simulink model "SFusion"  (Simulink 9.2)
settings: Solver=FixedStepAuto  StartTime=0.0  StopTime=inf  FixedStep=0.01  RelTol=1e-3  EnableMultiTasking=on
values from neighbouring files (symbols this model uses):
  CLOCK_SEL_PLL = uint8(hex2dec('01'))    [Sfusion.m]
  PWR_MGMNT_1 = uint8(hex2dec('6B'))    [Sfusion.m]
undefined symbols (not defined in the file or in its folder): BIT_H_RESET, BITS_DLPF_CFG_188HZ, BITS_FS_250DPS, BITS_FS_2G, Init, Initialize, MPUREG_ACCEL_CONFIG, MPUREG_GYRO_CONFIG, MPUREG_GYRO_XOUT_H, READ_FLAG
libraries: mbedblockslib x22, arduinolib x20, simulink x15
settings Model: Creator=Syed Imtiaz Ali Shah  LastModifiedBy=Syed Imtiaz Ali Shah  SimulationMode=external  ExtModeTrigDuration=2
settings DataIOCC: LimitDataPoints=off  SaveFormat=Dataset  SignalLoggingSaveFormat=Dataset
settings OptimizationCC: EnhancedBackFolding=on  PassReuseOutputArgsAs=Individual arguments  LifeSpan=auto  MaxStackSize=64  OptimizeBlockOrder=speed  DifferentSizesBufferReuse=on  OptimizationCustomize=off
settings DebuggingCC: UnderspecifiedInitializationDetection=Simplified  MergeDetectMultiDrivingBlocksExec=error  ParameterTunabilityLossMsg=error  FcnCallInpInsideContextMsg=error  StateNameClashWarn=none  SFUnexpectedBacktrackingDiag=error  SFNoUnconditionalDefaultTransitionDiag=error  SFExecutionAtInitializationDiag=warning
settings HardwareCC: ProdBitPerInt=16  ProdBitPerPointer=16  ProdBitPerSizeT=16  ProdBitPerPtrDiffT=16  ProdIntDivRoundTo=Zero  ProdEndianess=LittleEndian  ProdWordSize=8  ProdHWDeviceType=Atmel->AVR
settings ModelReferenceCC: PropagateSignalLabelsOutOfModel=on
settings SFSimCC: SimUseLocalCustomCode=on  MATLABDynamicMemAlloc=off
settings RTWCC: SystemTargetFile=ert.tlc  HardwareBoard=Arduino Mega 2560  TLCOptions=-aInlineSetEventsForThisBaseRateFcn=TLC_FALSE -aSuppressMultiTaskScheduler=TLC_FALSE -aRateBasedStepFcn=1  TemplateMakefile=ert_default_tmf  Description=Embedded Coder  GenerateReport=on  RTWUseLocalCustomCode=on  Toolchain=Arduino AVR  BuildConfiguration=Faster Runs  IncludeHyperlinkInReport=on  LaunchReport=on  GenerateTraceInfo=on  GenerateTraceReport=on  GenerateTraceReportSl=on  GenerateTraceReportSf=on  GenerateTraceReportEml=on
settings MATStruct: className=codertarget.tools.BuildHook  argsTopModelOnly=[]  excludedModels=[]  includeReferencedModels=on  includeTopModel=on  enabled=on  UseCoderTarget=[1]  TargetHardware=Arduino Mega 2560  RTOS=Baremetal  Scheduler_interrupt_source=[0.0]  DataVersion=2016.02  IPAddress=codertarget.arduinobase.registry.getLoopbackIP;  Port=17725  Verbose=[0]  Configuration=Serial  COMPortBaud=921600  BuildAction=Build, load and run  Set_host_COM_port=Manually  COM_port_number=4  Enable_SimulinkIO=[1.0]  Enable_overrun_detection=[0.0]  Digital_output_to_set_on_overrun=13  Analog_input_reference_voltage=[0.0]  Serial0_baud_rate=9600  Serial1_baud_rate=9600  Serial2_baud_rate=9600  Serial3_baud_rate=9600  I2C0BusSpeedHz=100000  SPI_clock_out_frequency=1000  SPI_mode=Mode 0 - Clock Polarity 0, Clock Phase 0  SPI_bitorder=MSB first  Disable_DHCP_Ethernet=[0.0]  Local_ip_address=192.168.0.20  Local_mac_address=DE:AD:BE:EF:FE:ED  Wifi_Hardware=WiFi shield  Disable_DHCP_Wifi=[0.0]  Wifi_ip_address=192.168.1.20  Wifi_SSID=yourNetwork  Set_Wifi_Encryption=None  Wifi_WEP_key=D0D0DEADF00DABBADEAFBEADED  Wifi_WEP_key_index=0  Wifi_WPA_password=secretPassword  Wifi_ESP8266_HW_serial_port=Serial 0  Enable_CustomServer=0  IP_address=184.106.153.149
settings CodeAppCC: ForceParamTrailComments=on  IgnoreCustomStorageClasses=off  OperatorAnnotations=on  SimulinkDataObjDesc=on  SFDataObjDesc=on  InsertBlockDesc=on  StateflowObjectComments=off
settings ERTTargetCC: SupportContinuousTime=on  SupportVariableSizeSignals=on
settings ConfigComp: CovMetricSettings=dwe  CovHtmlReporting=off  CovSaveCumulativeToWorkspaceVar=off  CovSaveSingleToWorkspaceVar=off  CovExternalEMLEnable=on

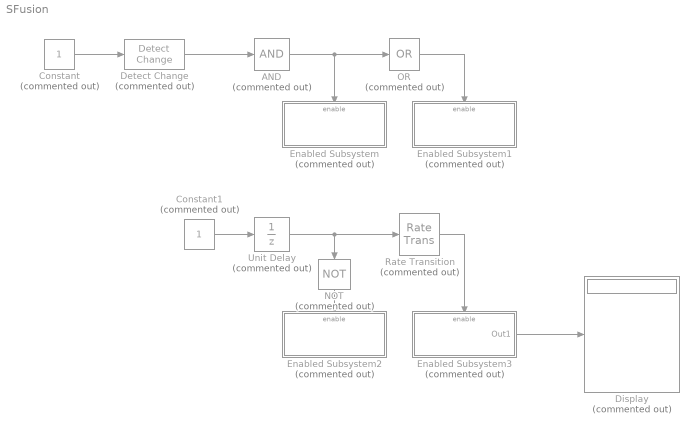
== system SFusion ==
  AND : Logic  Commented=on  Inputs=1  AllPortsSameDT=off  OutDataTypeStr=boolean
  Constant : Constant  Commented=on
  Constant1 : Constant  Commented=on
  Detect Change : simulink/Logic and Bit Operations/Detect Change  Commented=on  vinit=0  OutDataTypeStr=boolean
  Display : Display  Commented=on
  Enabled Subsystem : Subsystem  Commented=on  TreatAsAtomicUnit=on
  Enabled Subsystem1 : Subsystem  Commented=on  TreatAsAtomicUnit=on
  Enabled Subsystem2 : Subsystem  Commented=on  TreatAsAtomicUnit=on
  Enabled Subsystem3 : Subsystem  Commented=on  TreatAsAtomicUnit=on
  NOT : Logic  Commented=on  Operator=NOT  AllPortsSameDT=off  OutDataTypeStr=boolean
  OR : Logic  Commented=on  Operator=OR  Inputs=1  AllPortsSameDT=off  OutDataTypeStr=boolean
  Rate Transition : RateTransition  Commented=on
  Unit Delay : UnitDelay  Commented=on  SampleTime=-1
  wires:
  Constant/1 -> Detect Change/1
  Detect Change/1 -> AND/1
  AND/1 -> OR/1, Enabled Subsystem/Enable
  OR/1 -> Enabled Subsystem1/Enable
  Constant1/1 -> Unit Delay/1
  NOT/1 -> Enabled Subsystem2/Enable
  Unit Delay/1 -> NOT/1, Rate Transition/1
  Rate Transition/1 -> Enabled Subsystem3/Enable
  Enabled Subsystem3/1(Out1) -> Display/1

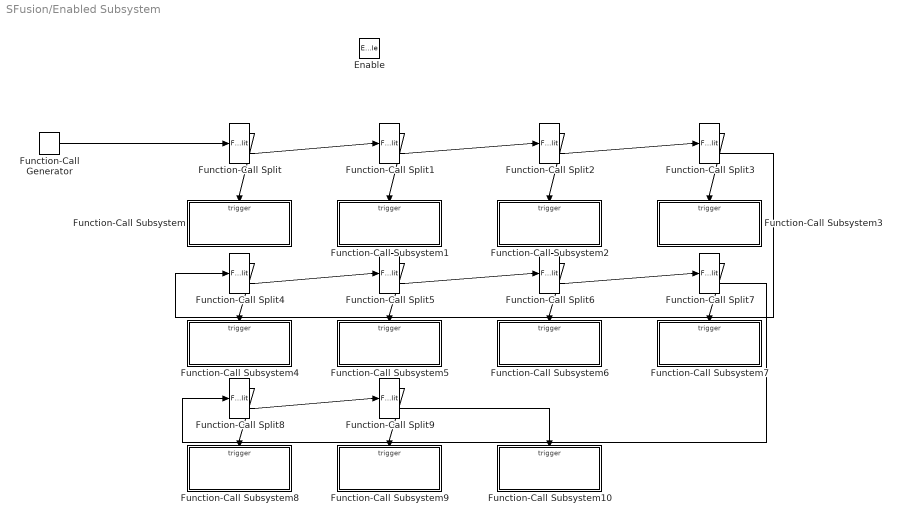
== system SFusion/Enabled Subsystem ==
  Enable : EnablePort
  Function-Call Generator : simulink/Ports & Subsystems/Function-Call Generator  sample_time=1  numberOfIterations=1
  Function-Call Split{,1..9} (10 alike) : FunctionCallSplit  NumOutputPorts=2
  Function-Call Subsystem : Subsystem  TreatAsAtomicUnit=on
  Function-Call Subsystem1 : Subsystem  TreatAsAtomicUnit=on
  Function-Call Subsystem10 : Subsystem  TreatAsAtomicUnit=on
  Function-Call Subsystem2 : Subsystem  TreatAsAtomicUnit=on
  Function-Call Subsystem3 : Subsystem  TreatAsAtomicUnit=on
  Function-Call Subsystem4 : Subsystem  TreatAsAtomicUnit=on
  Function-Call Subsystem5 : Subsystem  TreatAsAtomicUnit=on
  Function-Call Subsystem6 : Subsystem  TreatAsAtomicUnit=on
  Function-Call Subsystem7 : Subsystem  TreatAsAtomicUnit=on
  Function-Call Subsystem8 : Subsystem  TreatAsAtomicUnit=on
  Function-Call Subsystem9 : Subsystem  TreatAsAtomicUnit=on
  wires:
  Function-Call Split/1 -> Function-Call Subsystem/Trigger
  Function-Call Split/2 -> Function-Call Split1/1
  Function-Call Split7/1 -> Function-Call Subsystem7/Trigger
  Function-Call Split8/1 -> Function-Call Subsystem8/Trigger
  Function-Call Split9/2 -> Function-Call Subsystem10/Trigger
  Function-Call Split8/2 -> Function-Call Split9/1
  Function-Call Split9/1 -> Function-Call Subsystem9/Trigger
  Function-Call Split5/2 -> Function-Call Split6/1
  Function-Call Split6/1 -> Function-Call Subsystem6/Trigger
  Function-Call Split5/1 -> Function-Call Subsystem5/Trigger
  Function-Call Split4/1 -> Function-Call Subsystem4/Trigger
  Function-Call Split4/2 -> Function-Call Split5/1
  Function-Call Split3/2 -> Function-Call Split4/1
  Function-Call Split6/2 -> Function-Call Split7/1
  Function-Call Split7/2 -> Function-Call Split8/1
  Function-Call Split1/1 -> Function-Call Subsystem1/Trigger
  Function-Call Split1/2 -> Function-Call Split2/1
  Function-Call Split2/1 -> Function-Call Subsystem2/Trigger
  Function-Call Split2/2 -> Function-Call Split3/1
  Function-Call Split3/1 -> Function-Call Subsystem3/Trigger
  Function-Call Generator/1 -> Function-Call Split/1

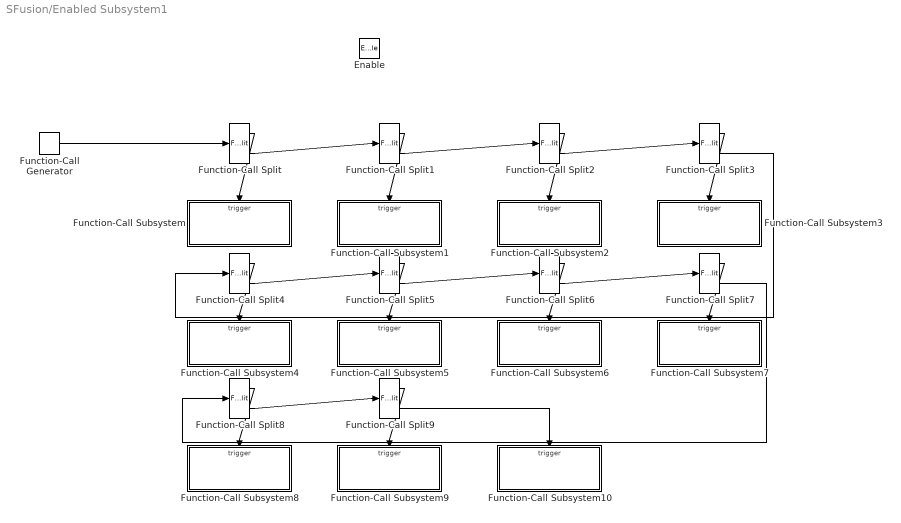
== system SFusion/Enabled Subsystem1 ==
  Enable : EnablePort
  Function-Call Generator : simulink/Ports & Subsystems/Function-Call Generator  sample_time=1  numberOfIterations=1
  Function-Call Split{,1..9} (10 alike) : FunctionCallSplit  NumOutputPorts=2
  Function-Call Subsystem : Subsystem  TreatAsAtomicUnit=on
  Function-Call Subsystem1 : Subsystem  TreatAsAtomicUnit=on
  Function-Call Subsystem10 : Subsystem  TreatAsAtomicUnit=on
  Function-Call Subsystem2 : Subsystem  TreatAsAtomicUnit=on
  Function-Call Subsystem3 : Subsystem  TreatAsAtomicUnit=on
  Function-Call Subsystem4 : Subsystem  TreatAsAtomicUnit=on
  Function-Call Subsystem5 : Subsystem  TreatAsAtomicUnit=on
  Function-Call Subsystem6 : Subsystem  TreatAsAtomicUnit=on
  Function-Call Subsystem7 : Subsystem  TreatAsAtomicUnit=on
  Function-Call Subsystem8 : Subsystem  TreatAsAtomicUnit=on
  Function-Call Subsystem9 : Subsystem  TreatAsAtomicUnit=on
  wires:
  Function-Call Generator/1 -> Function-Call Split/1
  Function-Call Split3/1 -> Function-Call Subsystem3/Trigger
  Function-Call Split2/2 -> Function-Call Split3/1
  Function-Call Split2/1 -> Function-Call Subsystem2/Trigger
  Function-Call Split1/2 -> Function-Call Split2/1
  Function-Call Split1/1 -> Function-Call Subsystem1/Trigger
  Function-Call Split7/2 -> Function-Call Split8/1
  Function-Call Split6/2 -> Function-Call Split7/1
  Function-Call Split3/2 -> Function-Call Split4/1
  Function-Call Split4/2 -> Function-Call Split5/1
  Function-Call Split4/1 -> Function-Call Subsystem4/Trigger
  Function-Call Split5/1 -> Function-Call Subsystem5/Trigger
  Function-Call Split6/1 -> Function-Call Subsystem6/Trigger
  Function-Call Split5/2 -> Function-Call Split6/1
  Function-Call Split9/1 -> Function-Call Subsystem9/Trigger
  Function-Call Split8/2 -> Function-Call Split9/1
  Function-Call Split9/2 -> Function-Call Subsystem10/Trigger
  Function-Call Split8/1 -> Function-Call Subsystem8/Trigger
  Function-Call Split7/1 -> Function-Call Subsystem7/Trigger
  Function-Call Split/2 -> Function-Call Split1/1
  Function-Call Split/1 -> Function-Call Subsystem/Trigger

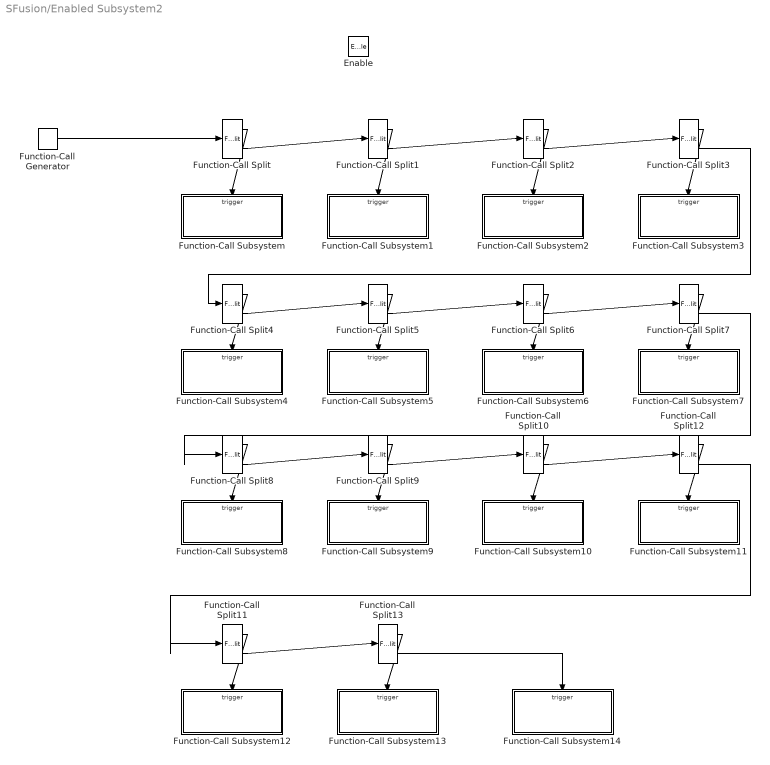
== system SFusion/Enabled Subsystem2 ==
  Enable : EnablePort
  Function-Call Generator : simulink/Ports & Subsystems/Function-Call Generator  sample_time=1  numberOfIterations=1
  Function-Call Split{,1..13} (14 alike) : FunctionCallSplit  NumOutputPorts=2
  Function-Call Subsystem : Subsystem  TreatAsAtomicUnit=on
  Function-Call Subsystem1 : Subsystem  TreatAsAtomicUnit=on
  Function-Call Subsystem10 : Subsystem  TreatAsAtomicUnit=on
  Function-Call Subsystem11 : Subsystem  TreatAsAtomicUnit=on
  Function-Call Subsystem12 : Subsystem  TreatAsAtomicUnit=on
  Function-Call Subsystem13 : Subsystem  TreatAsAtomicUnit=on
  Function-Call Subsystem14 : Subsystem  TreatAsAtomicUnit=on
  Function-Call Subsystem2 : Subsystem  TreatAsAtomicUnit=on
  Function-Call Subsystem3 : Subsystem  TreatAsAtomicUnit=on
  Function-Call Subsystem4 : Subsystem  TreatAsAtomicUnit=on
  Function-Call Subsystem5 : Subsystem  TreatAsAtomicUnit=on
  Function-Call Subsystem6 : Subsystem  TreatAsAtomicUnit=on
  Function-Call Subsystem7 : Subsystem  TreatAsAtomicUnit=on
  Function-Call Subsystem8 : Subsystem  TreatAsAtomicUnit=on
  Function-Call Subsystem9 : Subsystem  TreatAsAtomicUnit=on
  wires:
  Function-Call Generator/1 -> Function-Call Split/1
  Function-Call Split3/1 -> Function-Call Subsystem3/Trigger
  Function-Call Split2/2 -> Function-Call Split3/1
  Function-Call Split2/1 -> Function-Call Subsystem2/Trigger
  Function-Call Split1/2 -> Function-Call Split2/1
  Function-Call Split1/1 -> Function-Call Subsystem1/Trigger
  Function-Call Split7/2 -> Function-Call Split8/1
  Function-Call Split6/2 -> Function-Call Split7/1
  Function-Call Split3/2 -> Function-Call Split4/1
  Function-Call Split4/2 -> Function-Call Split5/1
  Function-Call Split4/1 -> Function-Call Subsystem4/Trigger
  Function-Call Split5/1 -> Function-Call Subsystem5/Trigger
  Function-Call Split6/1 -> Function-Call Subsystem6/Trigger
  Function-Call Split5/2 -> Function-Call Split6/1
  Function-Call Split9/1 -> Function-Call Subsystem9/Trigger
  Function-Call Split8/2 -> Function-Call Split9/1
  Function-Call Split8/1 -> Function-Call Subsystem8/Trigger
  Function-Call Split7/1 -> Function-Call Subsystem7/Trigger
  Function-Call Split/2 -> Function-Call Split1/1
  Function-Call Split/1 -> Function-Call Subsystem/Trigger
  Function-Call Split9/2 -> Function-Call Split10/1
  Function-Call Split10/1 -> Function-Call Subsystem10/Trigger
  Function-Call Split11/1 -> Function-Call Subsystem12/Trigger
  Function-Call Split12/1 -> Function-Call Subsystem11/Trigger
  Function-Call Split10/2 -> Function-Call Split12/1
  Function-Call Split12/2 -> Function-Call Split11/1
  Function-Call Split11/2 -> Function-Call Split13/1
  Function-Call Split13/1 -> Function-Call Subsystem13/Trigger
  Function-Call Split13/2 -> Function-Call Subsystem14/Trigger

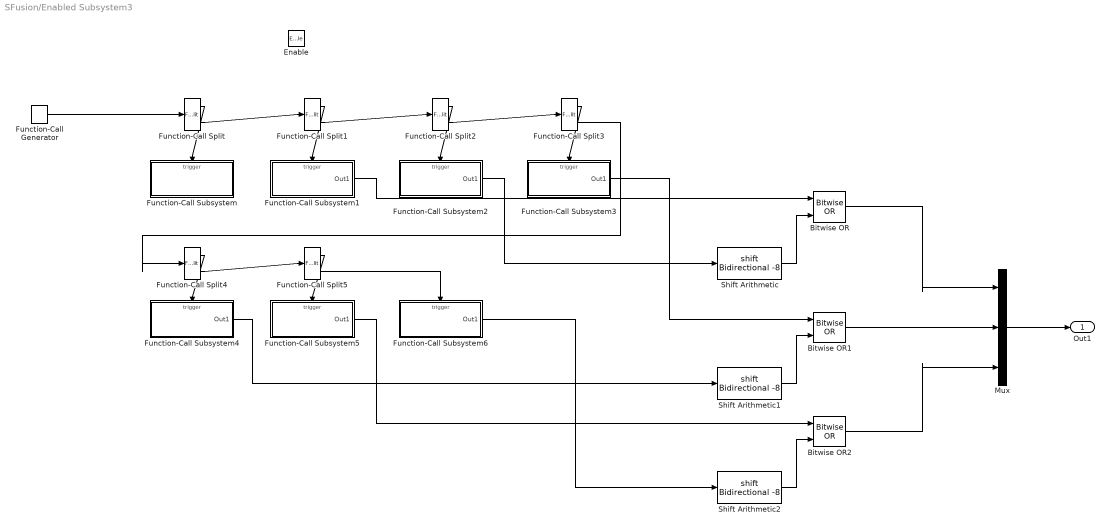
== system SFusion/Enabled Subsystem3 ==
  Enable : EnablePort
  Bitwise OR : simulink/Logic and Bit Operations/Bitwise Operator  logicop=OR  UseBitMask=off  NumInputPorts=2  BitMask=bin2dec('11011001')  BitMaskRealWorld=Stored Integer
  Bitwise OR1 : simulink/Logic and Bit Operations/Bitwise Operator  logicop=OR  UseBitMask=off  NumInputPorts=2  BitMask=bin2dec('11011001')  BitMaskRealWorld=Stored Integer
  Bitwise OR2 : simulink/Logic and Bit Operations/Bitwise Operator  logicop=OR  UseBitMask=off  NumInputPorts=2  BitMask=bin2dec('11011001')  BitMaskRealWorld=Stored Integer
  Function-Call Generator : simulink/Ports & Subsystems/Function-Call Generator  sample_time=1  numberOfIterations=1
  Function-Call Split{,1..5} (6 alike) : FunctionCallSplit  NumOutputPorts=2
  Function-Call Subsystem : Subsystem  TreatAsAtomicUnit=on
  Function-Call Subsystem1 : Subsystem  TreatAsAtomicUnit=on
  Function-Call Subsystem2 : Subsystem  TreatAsAtomicUnit=on
  Function-Call Subsystem3 : Subsystem  TreatAsAtomicUnit=on
  Function-Call Subsystem4 : Subsystem  TreatAsAtomicUnit=on
  Function-Call Subsystem5 : Subsystem  TreatAsAtomicUnit=on
  Function-Call Subsystem6 : Subsystem  TreatAsAtomicUnit=on
  Mux : Mux  Inputs=3
  Shift Arithmetic : ArithShift  BitShiftNumber=-8
  Shift Arithmetic1 : ArithShift  BitShiftNumber=-8
  Shift Arithmetic2 : ArithShift  BitShiftNumber=-8
  Out1 : Outport
  wires:
  Function-Call Split/1 -> Function-Call Subsystem/Trigger
  Function-Call Split/2 -> Function-Call Split1/1
  Function-Call Split5/2 -> Function-Call Subsystem6/Trigger
  Function-Call Split5/1 -> Function-Call Subsystem5/Trigger
  Function-Call Split4/1 -> Function-Call Subsystem4/Trigger
  Function-Call Split4/2 -> Function-Call Split5/1
  Function-Call Split1/1 -> Function-Call Subsystem1/Trigger
  Function-Call Split1/2 -> Function-Call Split2/1
  Function-Call Split2/1 -> Function-Call Subsystem2/Trigger
  Function-Call Split2/2 -> Function-Call Split3/1
  Function-Call Split3/1 -> Function-Call Subsystem3/Trigger
  Function-Call Generator/1 -> Function-Call Split/1
  Function-Call Split3/2 -> Function-Call Split4/1
  Function-Call Subsystem2/1(Out1) -> Shift Arithmetic/1
  Function-Call Subsystem1/1(Out1) -> Bitwise OR/1
  Shift Arithmetic/1 -> Bitwise OR/2
  Shift Arithmetic1/1 -> Bitwise OR1/2
  Function-Call Subsystem3/1(Out1) -> Bitwise OR1/1
  Function-Call Subsystem4/1(Out1) -> Shift Arithmetic1/1
  Shift Arithmetic2/1 -> Bitwise OR2/2
  Function-Call Subsystem5/1(Out1) -> Bitwise OR2/1
  Function-Call Subsystem6/1(Out1) -> Shift Arithmetic2/1
  Bitwise OR1/1 -> Mux/2
  Bitwise OR/1 -> Mux/1
  Bitwise OR2/1 -> Mux/3
  Mux/1 -> Out1/1

== system SFusion/Enabled Subsystem/Function-Call Subsystem ==
  function : TriggerPort  TriggerType=function-call  VariantControl=Variant
  Constant : Constant  Value=BIT_H_RESET
  SPI Register Write : mbedblockslib/SPI Register Write  SPIModule=1  Mode=Master  BusSpeed=uint32( 1000000 )  Pin=7  FirstBitToTransfer=Most significant bit (MSB)  ClockMode=0  BlockFunction=Write  RegisterAddress=MPUREG_PWR_MGMT_1  OutputDataType=int8  OutputDataLength=1  UseCustomSSPin=Explicit GPIO calls  ActiveLowSSPin=Active low
      settings: SourceProductName=Simulink Coder Support Package for BBC microbit Board  SourceProductBaseCode=MICROBIT
  wires:
  Constant/1 -> SPI Register Write/1

== system SFusion/Enabled Subsystem/Function-Call Subsystem1 ==
  function : TriggerPort  TriggerType=function-call  VariantControl=Variant
  Constant : Constant
  SPI Register Write : mbedblockslib/SPI Register Write  SPIModule=1  Mode=Master  BusSpeed=uint32( 1000000 )  Pin=7  FirstBitToTransfer=Most significant bit (MSB)  ClockMode=0  BlockFunction=Write  RegisterAddress=MPUREG_PWR_MGMT_1  OutputDataType=int8  OutputDataLength=1  UseCustomSSPin=Explicit GPIO calls  ActiveLowSSPin=Active low
      settings: SourceProductName=Simulink Coder Support Package for BBC microbit Board  SourceProductBaseCode=MICROBIT
  wires:
  Constant/1 -> SPI Register Write/1

== system SFusion/Enabled Subsystem/Function-Call Subsystem10 ==
  function : TriggerPort  TriggerType=function-call  VariantControl=Variant
  Constant : Constant  Value=Initialize(11,1)
  SPI Register Write : mbedblockslib/SPI Register Write  SPIModule=1  Mode=Master  BusSpeed=uint32( 1000000 )  Pin=7  FirstBitToTransfer=Most significant bit (MSB)  ClockMode=0  BlockFunction=Write  RegisterAddress=Initialize(11,2)  OutputDataType=int8  OutputDataLength=1  UseCustomSSPin=Explicit GPIO calls  ActiveLowSSPin=Active low
      settings: SourceProductName=Simulink Coder Support Package for BBC microbit Board  SourceProductBaseCode=MICROBIT
  wires:
  Constant/1 -> SPI Register Write/1

== system SFusion/Enabled Subsystem/Function-Call Subsystem2 ==
  function : TriggerPort  TriggerType=function-call  VariantControl=Variant
  Constant : Constant  Value=0
  SPI Register Write : mbedblockslib/SPI Register Write  SPIModule=1  Mode=Master  BusSpeed=uint32( 1000000 )  Pin=7  FirstBitToTransfer=Most significant bit (MSB)  ClockMode=0  BlockFunction=Write  RegisterAddress=MPUREG_PWR_MGMT_2  OutputDataType=int8  OutputDataLength=1  UseCustomSSPin=Explicit GPIO calls  ActiveLowSSPin=Active low
      settings: SourceProductName=Simulink Coder Support Package for BBC microbit Board  SourceProductBaseCode=MICROBIT
  wires:
  Constant/1 -> SPI Register Write/1

== system SFusion/Enabled Subsystem/Function-Call Subsystem3 ==
  function : TriggerPort  TriggerType=function-call  VariantControl=Variant
  Constant : Constant  Value=BITS_DLPF_CFG_188HZ
  SPI Register Write : mbedblockslib/SPI Register Write  SPIModule=1  Mode=Master  BusSpeed=uint32( 1000000 )  Pin=7  FirstBitToTransfer=Most significant bit (MSB)  ClockMode=0  BlockFunction=Write  RegisterAddress=MPUREG_CONFIG  OutputDataType=int8  OutputDataLength=1  UseCustomSSPin=Explicit GPIO calls  ActiveLowSSPin=Active low
      settings: SourceProductName=Simulink Coder Support Package for BBC microbit Board  SourceProductBaseCode=MICROBIT
  wires:
  Constant/1 -> SPI Register Write/1

== system SFusion/Enabled Subsystem/Function-Call Subsystem4 ==
  function : TriggerPort  TriggerType=function-call  VariantControl=Variant
  Constant : Constant  Value=Initialize(5,1)
  SPI Register Write : mbedblockslib/SPI Register Write  SPIModule=1  Mode=Master  BusSpeed=uint32( 1000000 )  Pin=7  FirstBitToTransfer=Most significant bit (MSB)  ClockMode=0  BlockFunction=Write  RegisterAddress=Initialize(5,2)  OutputDataType=int8  OutputDataLength=1  UseCustomSSPin=Explicit GPIO calls  ActiveLowSSPin=Active low
      settings: SourceProductName=Simulink Coder Support Package for BBC microbit Board  SourceProductBaseCode=MICROBIT
  wires:
  Constant/1 -> SPI Register Write/1

== system SFusion/Enabled Subsystem/Function-Call Subsystem5 ==
  function : TriggerPort  TriggerType=function-call  VariantControl=Variant
  Constant : Constant  Value=Initialize(6,1)
  SPI Register Write : mbedblockslib/SPI Register Write  SPIModule=1  Mode=Master  BusSpeed=uint32( 1000000 )  Pin=7  FirstBitToTransfer=Most significant bit (MSB)  ClockMode=0  BlockFunction=Write  RegisterAddress=Initialize(6,2)  OutputDataType=int8  OutputDataLength=1  UseCustomSSPin=Explicit GPIO calls  ActiveLowSSPin=Active low
      settings: SourceProductName=Simulink Coder Support Package for BBC microbit Board  SourceProductBaseCode=MICROBIT
  wires:
  Constant/1 -> SPI Register Write/1

== system SFusion/Enabled Subsystem/Function-Call Subsystem6 ==
  function : TriggerPort  TriggerType=function-call  VariantControl=Variant
  Constant : Constant  Value=Initialize(7,1)
  SPI Register Write : mbedblockslib/SPI Register Write  SPIModule=1  Mode=Master  BusSpeed=uint32( 1000000 )  Pin=7  FirstBitToTransfer=Most significant bit (MSB)  ClockMode=0  BlockFunction=Write  RegisterAddress=Initialize(7,2)  OutputDataType=int8  OutputDataLength=1  UseCustomSSPin=Explicit GPIO calls  ActiveLowSSPin=Active low
      settings: SourceProductName=Simulink Coder Support Package for BBC microbit Board  SourceProductBaseCode=MICROBIT
  wires:
  Constant/1 -> SPI Register Write/1

== system SFusion/Enabled Subsystem/Function-Call Subsystem7 ==
  function : TriggerPort  TriggerType=function-call  VariantControl=Variant
  Constant : Constant  Value=Initialize(8,1)
  SPI Register Write : mbedblockslib/SPI Register Write  SPIModule=1  Mode=Master  BusSpeed=uint32( 1000000 )  Pin=7  FirstBitToTransfer=Most significant bit (MSB)  ClockMode=0  BlockFunction=Write  RegisterAddress=Initialize(8,2)  OutputDataType=int8  OutputDataLength=1  UseCustomSSPin=Explicit GPIO calls  ActiveLowSSPin=Active low
      settings: SourceProductName=Simulink Coder Support Package for BBC microbit Board  SourceProductBaseCode=MICROBIT
  wires:
  Constant/1 -> SPI Register Write/1

== system SFusion/Enabled Subsystem/Function-Call Subsystem8 ==
  function : TriggerPort  TriggerType=function-call  VariantControl=Variant
  Constant : Constant  Value=Initialize(9,1)
  SPI Register Write : mbedblockslib/SPI Register Write  SPIModule=1  Mode=Master  BusSpeed=uint32( 1000000 )  Pin=7  FirstBitToTransfer=Most significant bit (MSB)  ClockMode=0  BlockFunction=Write  RegisterAddress=Initialize(9,2)  OutputDataType=int8  OutputDataLength=1  UseCustomSSPin=Explicit GPIO calls  ActiveLowSSPin=Active low
      settings: SourceProductName=Simulink Coder Support Package for BBC microbit Board  SourceProductBaseCode=MICROBIT
  wires:
  Constant/1 -> SPI Register Write/1

== system SFusion/Enabled Subsystem/Function-Call Subsystem9 ==
  function : TriggerPort  TriggerType=function-call  VariantControl=Variant
  Constant : Constant  Value=Initialize(10,1)
  SPI Register Write : mbedblockslib/SPI Register Write  SPIModule=1  Mode=Master  BusSpeed=uint32( 1000000 )  Pin=7  FirstBitToTransfer=Most significant bit (MSB)  ClockMode=0  BlockFunction=Write  RegisterAddress=Initialize(10,2)  OutputDataType=int8  OutputDataLength=1  UseCustomSSPin=Explicit GPIO calls  ActiveLowSSPin=Active low
      settings: SourceProductName=Simulink Coder Support Package for BBC microbit Board  SourceProductBaseCode=MICROBIT
  wires:
  Constant/1 -> SPI Register Write/1

== system SFusion/Enabled Subsystem1/Function-Call Subsystem ==
  function : TriggerPort  TriggerType=function-call  VariantControl=Variant
  Constant : Constant  Value=BIT_H_RESET
  SPI Register Write : mbedblockslib/SPI Register Write  SPIModule=1  Mode=Master  BusSpeed=uint32( 1000000 )  Pin=7  FirstBitToTransfer=Most significant bit (MSB)  ClockMode=0  BlockFunction=Write  RegisterAddress=MPUREG_PWR_MGMT_1  OutputDataType=int8  OutputDataLength=1  UseCustomSSPin=Explicit GPIO calls  ActiveLowSSPin=Active low
      settings: SourceProductName=Simulink Coder Support Package for BBC microbit Board  SourceProductBaseCode=MICROBIT
  wires:
  Constant/1 -> SPI Register Write/1

== system SFusion/Enabled Subsystem1/Function-Call Subsystem1 ==
  function : TriggerPort  TriggerType=function-call  VariantControl=Variant
  Constant : Constant
  SPI Register Write : mbedblockslib/SPI Register Write  SPIModule=1  Mode=Master  BusSpeed=uint32( 1000000 )  Pin=7  FirstBitToTransfer=Most significant bit (MSB)  ClockMode=0  BlockFunction=Write  RegisterAddress=MPUREG_PWR_MGMT_1  OutputDataType=int8  OutputDataLength=1  UseCustomSSPin=Explicit GPIO calls  ActiveLowSSPin=Active low
      settings: SourceProductName=Simulink Coder Support Package for BBC microbit Board  SourceProductBaseCode=MICROBIT
  wires:
  Constant/1 -> SPI Register Write/1

== system SFusion/Enabled Subsystem1/Function-Call Subsystem10 ==
  function : TriggerPort  TriggerType=function-call  VariantControl=Variant
  Constant : Constant  Value=Initialize(11,1)
  SPI Register Write : mbedblockslib/SPI Register Write  SPIModule=1  Mode=Master  BusSpeed=uint32( 1000000 )  Pin=7  FirstBitToTransfer=Most significant bit (MSB)  ClockMode=0  BlockFunction=Write  RegisterAddress=Initialize(11,2)  OutputDataType=int8  OutputDataLength=1  UseCustomSSPin=Explicit GPIO calls  ActiveLowSSPin=Active low
      settings: SourceProductName=Simulink Coder Support Package for BBC microbit Board  SourceProductBaseCode=MICROBIT
  wires:
  Constant/1 -> SPI Register Write/1

== system SFusion/Enabled Subsystem1/Function-Call Subsystem2 ==
  function : TriggerPort  TriggerType=function-call  VariantControl=Variant
  Constant : Constant  Value=0
  SPI Register Write : mbedblockslib/SPI Register Write  SPIModule=1  Mode=Master  BusSpeed=uint32( 1000000 )  Pin=7  FirstBitToTransfer=Most significant bit (MSB)  ClockMode=0  BlockFunction=Write  RegisterAddress=MPUREG_PWR_MGMT_2  OutputDataType=int8  OutputDataLength=1  UseCustomSSPin=Explicit GPIO calls  ActiveLowSSPin=Active low
      settings: SourceProductName=Simulink Coder Support Package for BBC microbit Board  SourceProductBaseCode=MICROBIT
  wires:
  Constant/1 -> SPI Register Write/1

== system SFusion/Enabled Subsystem1/Function-Call Subsystem3 ==
  function : TriggerPort  TriggerType=function-call  VariantControl=Variant
  Constant : Constant  Value=BITS_DLPF_CFG_188HZ
  SPI Register Write : mbedblockslib/SPI Register Write  SPIModule=1  Mode=Master  BusSpeed=uint32( 1000000 )  Pin=7  FirstBitToTransfer=Most significant bit (MSB)  ClockMode=0  BlockFunction=Write  RegisterAddress=MPUREG_CONFIG  OutputDataType=int8  OutputDataLength=1  UseCustomSSPin=Explicit GPIO calls  ActiveLowSSPin=Active low
      settings: SourceProductName=Simulink Coder Support Package for BBC microbit Board  SourceProductBaseCode=MICROBIT
  wires:
  Constant/1 -> SPI Register Write/1

== system SFusion/Enabled Subsystem1/Function-Call Subsystem4 ==
  function : TriggerPort  TriggerType=function-call  VariantControl=Variant
  Constant : Constant  Value=Initialize(5,1)
  SPI Register Write : mbedblockslib/SPI Register Write  SPIModule=1  Mode=Master  BusSpeed=uint32( 1000000 )  Pin=7  FirstBitToTransfer=Most significant bit (MSB)  ClockMode=0  BlockFunction=Write  RegisterAddress=Initialize(5,2)  OutputDataType=int8  OutputDataLength=1  UseCustomSSPin=Explicit GPIO calls  ActiveLowSSPin=Active low
      settings: SourceProductName=Simulink Coder Support Package for BBC microbit Board  SourceProductBaseCode=MICROBIT
  wires:
  Constant/1 -> SPI Register Write/1

== system SFusion/Enabled Subsystem1/Function-Call Subsystem5 ==
  function : TriggerPort  TriggerType=function-call  VariantControl=Variant
  Constant : Constant  Value=Initialize(6,1)
  SPI Register Write : mbedblockslib/SPI Register Write  SPIModule=1  Mode=Master  BusSpeed=uint32( 1000000 )  Pin=7  FirstBitToTransfer=Most significant bit (MSB)  ClockMode=0  BlockFunction=Write  RegisterAddress=Initialize(6,2)  OutputDataType=int8  OutputDataLength=1  UseCustomSSPin=Explicit GPIO calls  ActiveLowSSPin=Active low
      settings: SourceProductName=Simulink Coder Support Package for BBC microbit Board  SourceProductBaseCode=MICROBIT
  wires:
  Constant/1 -> SPI Register Write/1

== system SFusion/Enabled Subsystem1/Function-Call Subsystem6 ==
  function : TriggerPort  TriggerType=function-call  VariantControl=Variant
  Constant : Constant  Value=Initialize(7,1)
  SPI Register Write : mbedblockslib/SPI Register Write  SPIModule=1  Mode=Master  BusSpeed=uint32( 1000000 )  Pin=7  FirstBitToTransfer=Most significant bit (MSB)  ClockMode=0  BlockFunction=Write  RegisterAddress=Initialize(7,2)  OutputDataType=int8  OutputDataLength=1  UseCustomSSPin=Explicit GPIO calls  ActiveLowSSPin=Active low
      settings: SourceProductName=Simulink Coder Support Package for BBC microbit Board  SourceProductBaseCode=MICROBIT
  wires:
  Constant/1 -> SPI Register Write/1

== system SFusion/Enabled Subsystem1/Function-Call Subsystem7 ==
  function : TriggerPort  TriggerType=function-call  VariantControl=Variant
  Constant : Constant  Value=Initialize(8,1)
  SPI Register Write : mbedblockslib/SPI Register Write  SPIModule=1  Mode=Master  BusSpeed=uint32( 1000000 )  Pin=7  FirstBitToTransfer=Most significant bit (MSB)  ClockMode=0  BlockFunction=Write  RegisterAddress=Initialize(8,2)  OutputDataType=int8  OutputDataLength=1  UseCustomSSPin=Explicit GPIO calls  ActiveLowSSPin=Active low
      settings: SourceProductName=Simulink Coder Support Package for BBC microbit Board  SourceProductBaseCode=MICROBIT
  wires:
  Constant/1 -> SPI Register Write/1

== system SFusion/Enabled Subsystem1/Function-Call Subsystem8 ==
  function : TriggerPort  TriggerType=function-call  VariantControl=Variant
  Constant : Constant  Value=Initialize(9,1)
  SPI Register Write : mbedblockslib/SPI Register Write  SPIModule=1  Mode=Master  BusSpeed=uint32( 1000000 )  Pin=7  FirstBitToTransfer=Most significant bit (MSB)  ClockMode=0  BlockFunction=Write  RegisterAddress=Initialize(9,2)  OutputDataType=int8  OutputDataLength=1  UseCustomSSPin=Explicit GPIO calls  ActiveLowSSPin=Active low
      settings: SourceProductName=Simulink Coder Support Package for BBC microbit Board  SourceProductBaseCode=MICROBIT
  wires:
  Constant/1 -> SPI Register Write/1

== system SFusion/Enabled Subsystem1/Function-Call Subsystem9 ==
  function : TriggerPort  TriggerType=function-call  VariantControl=Variant
  Constant : Constant  Value=Initialize(10,1)
  SPI Register Write : mbedblockslib/SPI Register Write  SPIModule=1  Mode=Master  BusSpeed=uint32( 1000000 )  Pin=7  FirstBitToTransfer=Most significant bit (MSB)  ClockMode=0  BlockFunction=Write  RegisterAddress=Initialize(10,2)  OutputDataType=int8  OutputDataLength=1  UseCustomSSPin=Explicit GPIO calls  ActiveLowSSPin=Active low
      settings: SourceProductName=Simulink Coder Support Package for BBC microbit Board  SourceProductBaseCode=MICROBIT
  wires:
  Constant/1 -> SPI Register Write/1

== system SFusion/Enabled Subsystem2/Function-Call Subsystem ==
  function : TriggerPort  TriggerType=function-call  VariantControl=Variant
  Constant : Constant  Value=[PWR_MGMNT_1 CLOCK_SEL_PLL]
  SPI WriteRead : arduinolib/SPI WriteRead  slaveSelectPin_=10  blockPlatform=arduino
      settings: SourceProductName=Simulink Support Package for Arduino Hardware  SourceProductBaseCode=ARDUINO
  wires:
  Constant/1 -> SPI WriteRead/1

== system SFusion/Enabled Subsystem2/Function-Call Subsystem1 ==
  function : TriggerPort  TriggerType=function-call  VariantControl=Variant
  Constant : Constant  Value=Init(2,:)
  SPI WriteRead : arduinolib/SPI WriteRead  slaveSelectPin_=10  blockPlatform=arduino
      settings: SourceProductName=Simulink Support Package for Arduino Hardware  SourceProductBaseCode=ARDUINO
  wires:
  Constant/1 -> SPI WriteRead/1

== system SFusion/Enabled Subsystem2/Function-Call Subsystem10 ==
  function : TriggerPort  TriggerType=function-call  VariantControl=Variant
  Constant : Constant  Value=Init(11,:)
  SPI WriteRead : arduinolib/SPI WriteRead  slaveSelectPin_=10  blockPlatform=arduino
      settings: SourceProductName=Simulink Support Package for Arduino Hardware  SourceProductBaseCode=ARDUINO
  wires:
  Constant/1 -> SPI WriteRead/1

== system SFusion/Enabled Subsystem2/Function-Call Subsystem11 ==
  function : TriggerPort  TriggerType=function-call  VariantControl=Variant
  System Outputs : Subsystem  mask(System Outputs){ShowInLibBrowser=0}
      mask prompts: ShowInLibBrowser "Simulink:masks:CustCodeMaskParam1_MP"
      settings: CopyFcn=cccopyfcn(gcb)  OpenFcn=ccopenfcn('System Outputs Function')
      mask Help: eval('feval(''rtwprivate'',''rtwhelpview'',''rtw_sys_outputs_block'')');
      mask Display: disp('System\nOutputs');

== system SFusion/Enabled Subsystem2/Function-Call Subsystem12 ==
  function : TriggerPort  TriggerType=function-call  VariantControl=Variant
  Constant : Constant  Value=[MPUREG_ACCEL_CONFIG BITS_FS_2G]
  Data Type Conversion : DataTypeConversion  OutDataTypeStr=uint8
  SPI WriteRead : arduinolib/SPI WriteRead  slaveSelectPin_=10  blockPlatform=arduino
      settings: SourceProductName=Simulink Support Package for Arduino Hardware  SourceProductBaseCode=ARDUINO
  wires:
  Constant/1 -> Data Type Conversion/1
  Data Type Conversion/1 -> SPI WriteRead/1

== system SFusion/Enabled Subsystem2/Function-Call Subsystem13 ==
  function : TriggerPort  TriggerType=function-call  VariantControl=Variant
  Constant : Constant  Value=[MPUREG_GYRO_CONFIG BITS_FS_250DPS]
  Data Type Conversion : DataTypeConversion  OutDataTypeStr=uint8
  SPI WriteRead : arduinolib/SPI WriteRead  slaveSelectPin_=10  blockPlatform=arduino
      settings: SourceProductName=Simulink Support Package for Arduino Hardware  SourceProductBaseCode=ARDUINO
  wires:
  Constant/1 -> Data Type Conversion/1
  Data Type Conversion/1 -> SPI WriteRead/1

== system SFusion/Enabled Subsystem2/Function-Call Subsystem14 ==
  function : TriggerPort  TriggerType=function-call  VariantControl=Variant
  System Outputs : Subsystem  mask(System Outputs){ShowInLibBrowser=0}
      mask prompts: ShowInLibBrowser "Simulink:masks:CustCodeMaskParam1_MP"
      settings: CopyFcn=cccopyfcn(gcb)  OpenFcn=ccopenfcn('System Outputs Function')
      mask Help: eval('feval(''rtwprivate'',''rtwhelpview'',''rtw_sys_outputs_block'')');
      mask Display: disp('System\nOutputs');

== system SFusion/Enabled Subsystem2/Function-Call Subsystem2 ==
  function : TriggerPort  TriggerType=function-call  VariantControl=Variant
  Constant : Constant  Value=Init(3,:)
  SPI WriteRead : arduinolib/SPI WriteRead  slaveSelectPin_=10  blockPlatform=arduino
      settings: SourceProductName=Simulink Support Package for Arduino Hardware  SourceProductBaseCode=ARDUINO
  wires:
  Constant/1 -> SPI WriteRead/1

== system SFusion/Enabled Subsystem2/Function-Call Subsystem3 ==
  function : TriggerPort  TriggerType=function-call  VariantControl=Variant
  Constant : Constant  Value=Init(4,:)
  SPI WriteRead : arduinolib/SPI WriteRead  slaveSelectPin_=10  blockPlatform=arduino
      settings: SourceProductName=Simulink Support Package for Arduino Hardware  SourceProductBaseCode=ARDUINO
  wires:
  Constant/1 -> SPI WriteRead/1

== system SFusion/Enabled Subsystem2/Function-Call Subsystem4 ==
  function : TriggerPort  TriggerType=function-call  VariantControl=Variant
  Constant : Constant  Value=Init(5,:)
  SPI WriteRead : arduinolib/SPI WriteRead  slaveSelectPin_=10  blockPlatform=arduino
      settings: SourceProductName=Simulink Support Package for Arduino Hardware  SourceProductBaseCode=ARDUINO
  wires:
  Constant/1 -> SPI WriteRead/1

== system SFusion/Enabled Subsystem2/Function-Call Subsystem5 ==
  function : TriggerPort  TriggerType=function-call  VariantControl=Variant
  Constant : Constant  Value=Init(6,:)
  SPI WriteRead : arduinolib/SPI WriteRead  slaveSelectPin_=10  blockPlatform=arduino
      settings: SourceProductName=Simulink Support Package for Arduino Hardware  SourceProductBaseCode=ARDUINO
  wires:
  Constant/1 -> SPI WriteRead/1

== system SFusion/Enabled Subsystem2/Function-Call Subsystem6 ==
  function : TriggerPort  TriggerType=function-call  VariantControl=Variant
  Constant : Constant  Value=Init(7,:)
  SPI WriteRead : arduinolib/SPI WriteRead  slaveSelectPin_=10  blockPlatform=arduino
      settings: SourceProductName=Simulink Support Package for Arduino Hardware  SourceProductBaseCode=ARDUINO
  wires:
  Constant/1 -> SPI WriteRead/1

== system SFusion/Enabled Subsystem2/Function-Call Subsystem7 ==
  function : TriggerPort  TriggerType=function-call  VariantControl=Variant
  Constant : Constant  Value=Init(8,:)
  SPI WriteRead : arduinolib/SPI WriteRead  slaveSelectPin_=10  blockPlatform=arduino
      settings: SourceProductName=Simulink Support Package for Arduino Hardware  SourceProductBaseCode=ARDUINO
  wires:
  Constant/1 -> SPI WriteRead/1

== system SFusion/Enabled Subsystem2/Function-Call Subsystem8 ==
  function : TriggerPort  TriggerType=function-call  VariantControl=Variant
  Constant : Constant  Value=Init(9,:)
  SPI WriteRead : arduinolib/SPI WriteRead  slaveSelectPin_=10  blockPlatform=arduino
      settings: SourceProductName=Simulink Support Package for Arduino Hardware  SourceProductBaseCode=ARDUINO
  wires:
  Constant/1 -> SPI WriteRead/1

== system SFusion/Enabled Subsystem2/Function-Call Subsystem9 ==
  function : TriggerPort  TriggerType=function-call  VariantControl=Variant
  Constant : Constant  Value=Init(10,:)
  SPI WriteRead : arduinolib/SPI WriteRead  slaveSelectPin_=10  blockPlatform=arduino
      settings: SourceProductName=Simulink Support Package for Arduino Hardware  SourceProductBaseCode=ARDUINO
  wires:
  Constant/1 -> SPI WriteRead/1

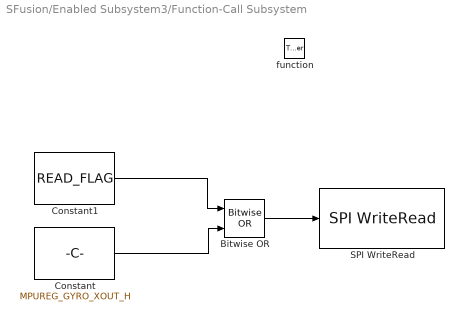
== system SFusion/Enabled Subsystem3/Function-Call Subsystem ==
  function : TriggerPort  TriggerType=function-call  VariantControl=Variant
  Bitwise OR : simulink/Logic and Bit Operations/Bitwise Operator  logicop=OR  UseBitMask=off  NumInputPorts=2  BitMask=bin2dec('11011001')  BitMaskRealWorld=Stored Integer
  Constant : Constant  Value=MPUREG_GYRO_XOUT_H  OutDataTypeStr=uint8
  Constant1 : Constant  Value=READ_FLAG  OutDataTypeStr=uint8
  SPI WriteRead : arduinolib/SPI WriteRead  slaveSelectPin_=10  blockPlatform=arduino
      settings: SourceProductName=Simulink Support Package for Arduino Hardware  SourceProductBaseCode=ARDUINO
  wires:
  Bitwise OR/1 -> SPI WriteRead/1
  Constant/1 -> Bitwise OR/2
  Constant1/1 -> Bitwise OR/1

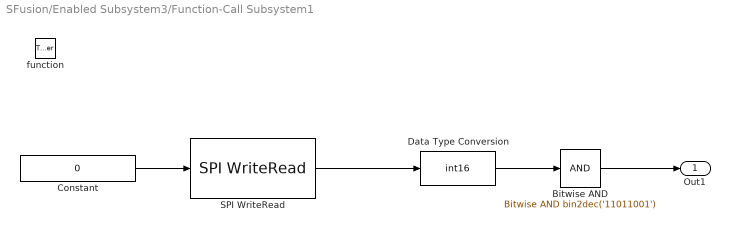
== system SFusion/Enabled Subsystem3/Function-Call Subsystem1 ==
  function : TriggerPort  TriggerType=function-call  VariantControl=Variant
  Bitwise AND : simulink/Logic and Bit Operations/Bitwise Operator  logicop=AND  UseBitMask=on  BitMask=bin2dec('11011001')  BitMaskRealWorld=Stored Integer
  Constant : Constant  Value=0  OutDataTypeStr=uint8
  Data Type Conversion : DataTypeConversion  OutDataTypeStr=int16
  SPI WriteRead : arduinolib/SPI WriteRead  slaveSelectPin_=10  blockPlatform=arduino
      settings: SourceProductName=Simulink Support Package for Arduino Hardware  SourceProductBaseCode=ARDUINO
  Out1 : Outport
  wires:
  Constant/1 -> SPI WriteRead/1
  SPI WriteRead/1 -> Data Type Conversion/1
  Data Type Conversion/1 -> Bitwise AND/1
  Bitwise AND/1 -> Out1/1

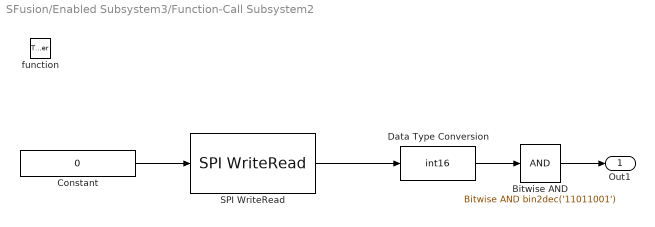
== system SFusion/Enabled Subsystem3/Function-Call Subsystem2 ==
  function : TriggerPort  TriggerType=function-call  VariantControl=Variant
  Bitwise AND : simulink/Logic and Bit Operations/Bitwise Operator  logicop=AND  UseBitMask=on  BitMask=bin2dec('11011001')  BitMaskRealWorld=Stored Integer
  Constant : Constant  Value=0  OutDataTypeStr=uint8
  Data Type Conversion : DataTypeConversion  OutDataTypeStr=int16
  SPI WriteRead : arduinolib/SPI WriteRead  slaveSelectPin_=10  blockPlatform=arduino
      settings: SourceProductName=Simulink Support Package for Arduino Hardware  SourceProductBaseCode=ARDUINO
  Out1 : Outport
  wires:
  SPI WriteRead/1 -> Data Type Conversion/1
  Constant/1 -> SPI WriteRead/1
  Data Type Conversion/1 -> Bitwise AND/1
  Bitwise AND/1 -> Out1/1

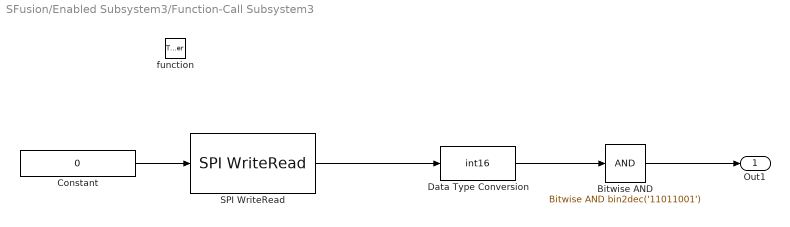
== system SFusion/Enabled Subsystem3/Function-Call Subsystem3 ==
  function : TriggerPort  TriggerType=function-call  VariantControl=Variant
  Bitwise AND : simulink/Logic and Bit Operations/Bitwise Operator  logicop=AND  UseBitMask=on  BitMask=bin2dec('11011001')  BitMaskRealWorld=Stored Integer
  Constant : Constant  Value=0  OutDataTypeStr=uint8
  Data Type Conversion : DataTypeConversion  OutDataTypeStr=int16
  SPI WriteRead : arduinolib/SPI WriteRead  slaveSelectPin_=10  blockPlatform=arduino
      settings: SourceProductName=Simulink Support Package for Arduino Hardware  SourceProductBaseCode=ARDUINO
  Out1 : Outport
  wires:
  SPI WriteRead/1 -> Data Type Conversion/1
  Constant/1 -> SPI WriteRead/1
  Data Type Conversion/1 -> Bitwise AND/1
  Bitwise AND/1 -> Out1/1

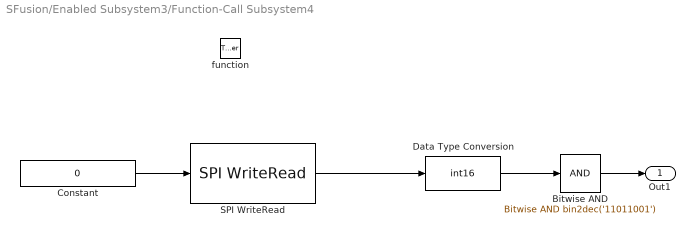
== system SFusion/Enabled Subsystem3/Function-Call Subsystem4 ==
  function : TriggerPort  TriggerType=function-call  VariantControl=Variant
  Bitwise AND : simulink/Logic and Bit Operations/Bitwise Operator  logicop=AND  UseBitMask=on  BitMask=bin2dec('11011001')  BitMaskRealWorld=Stored Integer
  Constant : Constant  Value=0  OutDataTypeStr=uint8
  Data Type Conversion : DataTypeConversion  OutDataTypeStr=int16
  SPI WriteRead : arduinolib/SPI WriteRead  slaveSelectPin_=10  blockPlatform=arduino
      settings: SourceProductName=Simulink Support Package for Arduino Hardware  SourceProductBaseCode=ARDUINO
  Out1 : Outport
  wires:
  SPI WriteRead/1 -> Data Type Conversion/1
  Constant/1 -> SPI WriteRead/1
  Data Type Conversion/1 -> Bitwise AND/1
  Bitwise AND/1 -> Out1/1

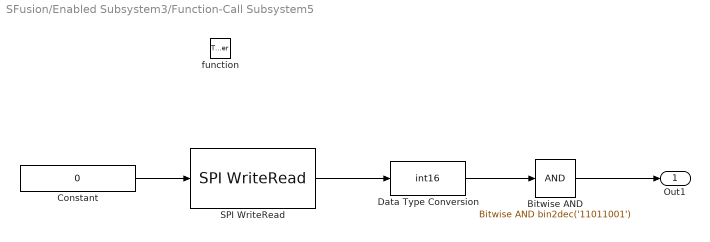
== system SFusion/Enabled Subsystem3/Function-Call Subsystem5 ==
  function : TriggerPort  TriggerType=function-call  VariantControl=Variant
  Bitwise AND : simulink/Logic and Bit Operations/Bitwise Operator  logicop=AND  UseBitMask=on  BitMask=bin2dec('11011001')  BitMaskRealWorld=Stored Integer
  Constant : Constant  Value=0  OutDataTypeStr=uint8
  Data Type Conversion : DataTypeConversion  OutDataTypeStr=int16
  SPI WriteRead : arduinolib/SPI WriteRead  slaveSelectPin_=10  blockPlatform=arduino
      settings: SourceProductName=Simulink Support Package for Arduino Hardware  SourceProductBaseCode=ARDUINO
  Out1 : Outport
  wires:
  SPI WriteRead/1 -> Data Type Conversion/1
  Constant/1 -> SPI WriteRead/1
  Data Type Conversion/1 -> Bitwise AND/1
  Bitwise AND/1 -> Out1/1

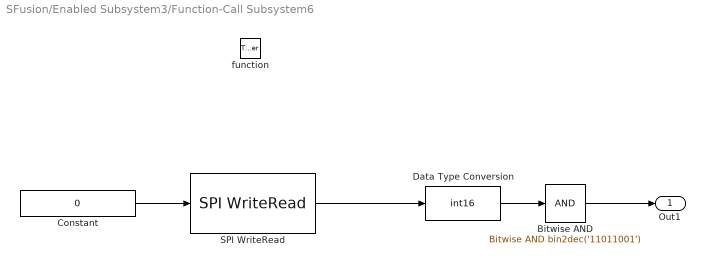
== system SFusion/Enabled Subsystem3/Function-Call Subsystem6 ==
  function : TriggerPort  TriggerType=function-call  VariantControl=Variant
  Bitwise AND : simulink/Logic and Bit Operations/Bitwise Operator  logicop=AND  UseBitMask=on  BitMask=bin2dec('11011001')  BitMaskRealWorld=Stored Integer
  Constant : Constant  Value=0  OutDataTypeStr=uint8
  Data Type Conversion : DataTypeConversion  OutDataTypeStr=int16
  SPI WriteRead : arduinolib/SPI WriteRead  slaveSelectPin_=10  blockPlatform=arduino
      settings: SourceProductName=Simulink Support Package for Arduino Hardware  SourceProductBaseCode=ARDUINO
  Out1 : Outport
  wires:
  SPI WriteRead/1 -> Data Type Conversion/1
  Constant/1 -> SPI WriteRead/1
  Data Type Conversion/1 -> Bitwise AND/1
  Bitwise AND/1 -> Out1/1

== system SFusion/Enabled Subsystem2/Function-Call Subsystem11/System Outputs ==

== system SFusion/Enabled Subsystem2/Function-Call Subsystem14/System Outputs ==
